simulink model "Sense_K_dth"  (R2016b)
settings: Solver=FixedStepAuto  StartTime=0.0  StopTime=tF  FixedStep=0.001  RelTol=1e-3
values from neighbouring files (symbols this model uses):
  K_dth = 0.05    [Proj_1b.m]    (also in Proj_5.m = -0.04; parameters.m = 0.05*sgn)
  M_d = M_d_r(i)    [Proj_7.m]    (also in parameters.m = 200*sgn)
  tau = tau_i(i)    [Proj_4.m]    (also in parameters.m = 0.05)
settings Model: Creator=Daniel  LastModifiedBy=Daniel

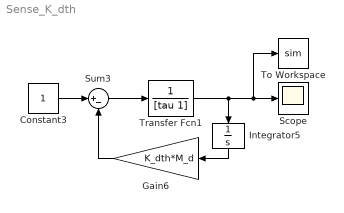
== system Sense_K_dth ==
  Constant3 : Constant
  Gain6 : Gain  Gain=K_dth*M_d
  Integrator5 : Integrator
  Scope : Scope
  Sum3 : Sum  Inputs=|+-
  To Workspace : ToWorkspace  VariableName=sim  SaveFormat=Timeseries  SampleTime=-1
  Transfer Fcn1 : TransferFcn  Denominator=[tau 1]
  wires:
  Sum3/1 -> Transfer Fcn1/1
  Transfer Fcn1/1 -> Scope/1, To Workspace/1, Integrator5/1
  Gain6/1 -> Sum3/2
  Integrator5/1 -> Gain6/1
  Constant3/1 -> Sum3/1
